simulink model "el_chem_25uA"  (R2024a)
settings: Solver=FixedStepDiscrete  StartTime=0.0  StopTime=inf  FixedStep=0.1  RelTol=1e-3
libraries: etargetslib x6, instrumentseriallib x3
settings Model: Creator=setm  LastModifiedBy=setm

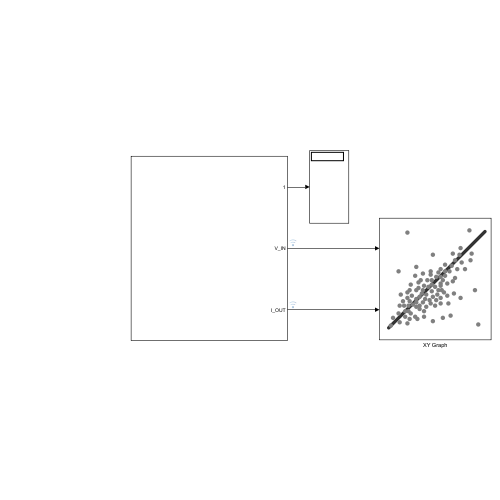
[thumbnail: Simulink's stored preview of the top-level diagram]
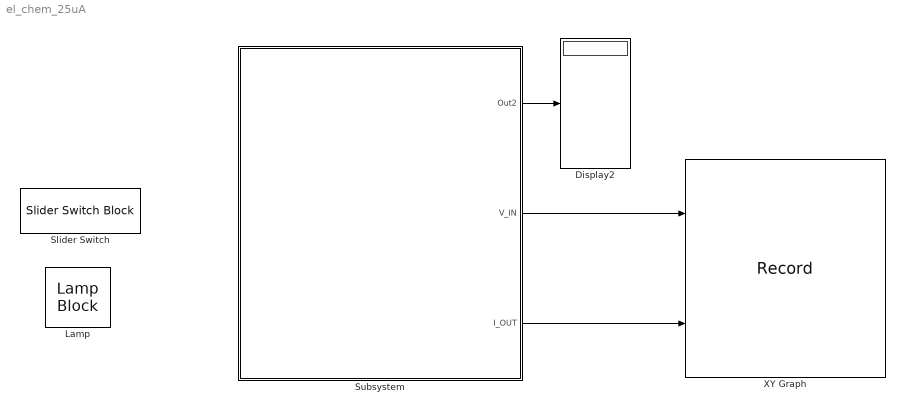
== system el_chem_25uA ==
  Display2 : Display
      settings: Decimation=5
  Lamp : LampBlock  LabelPosition=Hide
  Slider Switch : SliderSwitchBlock
      settings: Values={{'Off', 'On'}, [0 1]}
  Subsystem : Subsystem
  XY Graph : Record  FileSettingsInternal="{\"entries\":[{\"content\":{\"excelSettings\":{\"content\":{},\"type\":\"Streamout.ExcelSettings\"}},\"type\":\"Streamout.FileSettingStorage\",\"uuid\":\"\"}],\"packageUris\":[\"http:\\/\\/schema.mathworks.com\\/mf0\\/streamout_blocks\\/R2020a\"],\"version\":\"1.0\"}"  Layout=[1 1]  SignalsInternal="{\"entries\":[{\"content\":{\"signals\":[{\"content\":{\"blockPath\":[],\"dimensions\":[1],\"domain\":\"\",\"lineColor\":\"#a2142f\",\"plots\":[ 1 ],\"port\":1,\"signalID\":1,\"signalName\":\"Subsystem:2\"},\"type\":\"RecordBlkView.Signal\",\"uuid\":\"\"},{\"content\":{\"blockPath\":[],\"dimensions\":[1,1],\"domain\":\"\",\"lineColor\":\"#139fff\",\"plots\":[ 1 ],\"port\":2,\"signalID\":2,\"signalName\":\"Subsystem:3\"},\"type\":\"RecordBlkView.Signal\",\"uuid\":\"\"}]},\"type\":\"RecordBlkView.InputSignals\",\"uuid\":\"\"}],\"packageUris\":[\"http:\\/\\/schema.mathworks.com\\/mf0\\/streamout_blocks\\/R2020a\"],\"version\":\"1.0\"}"  VisualizationBindings="{\"xyplotplugin\":{\"info\":[{\"series\":[{\"bindingParametersList\":[{\"parameter\":\"X-Axis\",\"signalID\":1,\"signalName\":\"Subsystem:2\"},{\"parameter\":\"Y-Axis\",\"signalID\":2,\"signalName\":\"Subsystem:3\"}],\"seriesID\":0}],\"subplotID\":1}]}}"  CompatibilityTag=XY
  wires:
  Subsystem/1(Out2) -> Display2/1
  Subsystem/3(I_OUT) -> XY Graph/2
  Subsystem/2(V_IN) -> XY Graph/1

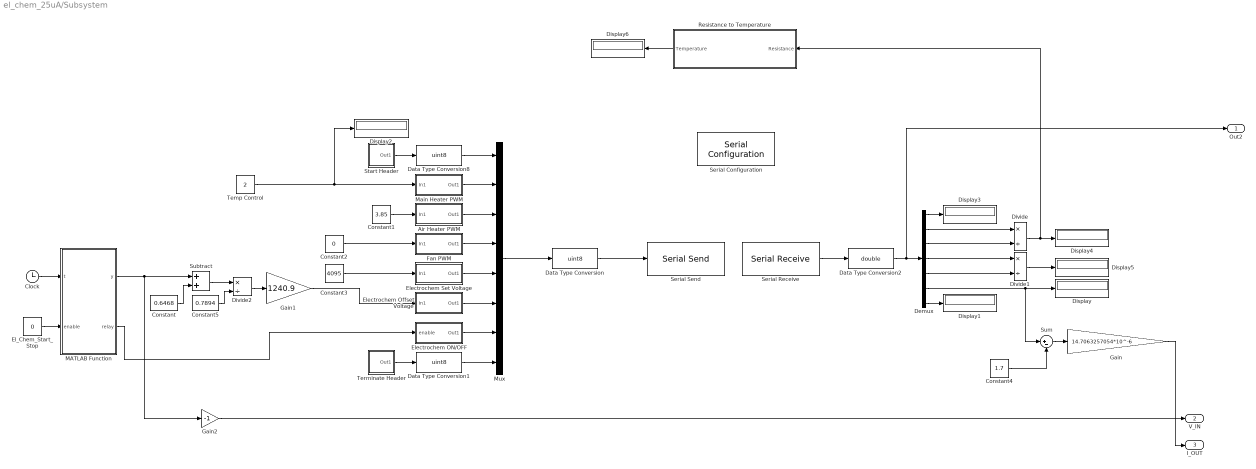
== system el_chem_25uA/Subsystem ==
  Air Heater PWM : Subsystem
  Clock : Clock
  Constant : Constant  Value=0.6468
  Constant1 : Constant  Value=3.85
  Constant2 : Constant  Value=0
  Constant3 : Constant  Value=4095
  Constant4 : Constant  Value=1.7
  Constant5 : Constant  Value=0.7894
  Data Type Conversion : DataTypeConversion  OutDataTypeStr=uint8  SaturateOnIntegerOverflow=off  RndMeth=Floor
  Data Type Conversion1 : DataTypeConversion  OutDataTypeStr=uint8  SaturateOnIntegerOverflow=off  RndMeth=Floor
  Data Type Conversion2 : DataTypeConversion  OutDataTypeStr=double  SaturateOnIntegerOverflow=off  RndMeth=Floor
  Data Type Conversion8 : DataTypeConversion  OutDataTypeStr=uint8  SaturateOnIntegerOverflow=off  RndMeth=Floor
  Demux : Demux  Outputs=7
  Display{,1..6} (7 alike) : Display
      Display1 settings: Decimation=5
      Display3 settings: Decimation=5
  Divide : Product  Inputs=*/
  Divide1 : Product  Inputs=*/
  Divide2 : Product  Inputs=*/
  El_Chem_Start_Stop : Constant  Value=0
  Electrochem ON/OFF : Subsystem
  Electrochem Offset Voltage : Subsystem
  Electrochem Set Voltage : Subsystem
  Fan PWM : Subsystem
  Gain : Gain  Gain=14.7063257054*10^-6
  Gain1 : Gain  Gain=1240.9
  Gain2 : Gain  Gain=-1
  MATLAB Function : MATLAB Function  TreatAsAtomicUnit=on
  Main Heater PWM : Subsystem
  Mux : Mux  Inputs=8
  Resistance to Temperature : Subsystem
  Serial Configuration : instrumentseriallib/Serial Configuration  Priority=-200000  PortSel=COM10  Port=COM10  ComPort=COM10  BaudRate=115200  DataBits=8  Parity=none  StopBits=1  ByteOrder=little-endian  FlowControl=none  Timeout=10  SimulateUsing=Interpreted execution  BlockInModel=on  aMode=1
  Serial Receive : instrumentseriallib/Serial Receive  Priority=1  PortSel=COM10  Port=COM10  ComPort=COM10  DataType=single  SaveDataType=uint8  ToggleHeader=off  Header=[]  ToggleDataSize=on  DataSize=[7 1]  ToggleTerminator=off  Terminator=<none>  CustomTerminator=[]  InputFormat=Column major  EnableBlockingMode=on  ActionDataUnavailable=Output last received value  ActionWhenDataUnavailable=Output last received value  CustomValue=0  SampleTime=0.1  SimulateUsing=Interpreted execution  BlockInModel=on  aMode=1
  Serial Send : instrumentseriallib/Serial Send  Priority=1  PortSel=COM10  Port=COM10  ComPort=COM10  Header=[]  Terminator=<none>  CustomTerminator=[]  EnableBlockingMode=on  SimulateUsing=Interpreted execution  BlockInModel=on  aMode=1
  Start Header : Subsystem
  Subtract : Sum
  Sum : Sum  Inputs=|+-
  Temp Control : Constant  Value=2
  Terminate Header : Subsystem
  Out2 : Outport
  V_IN : Outport  Port=2
  I_OUT : Outport  Port=3
  wires:
  Electrochem ON/OFF/1(Out1) -> Mux/7
  Constant2/1 -> Fan PWM/1(In1)
  Divide1/1 -> Display5/1
  Demux/7 -> Display1/1
  Demux/4 -> Divide1/1
  Demux/5 -> Divide1/2
  Mux/1 -> Data Type Conversion/1
  Data Type Conversion1/1 -> Mux/8
  Data Type Conversion8/1 -> Mux/1
  Data Type Conversion/1 -> Serial Send/1
  Air Heater PWM/1(Out1) -> Mux/3
  Demux/6 -> Sum/1, Display/1
  Constant1/1 -> Air Heater PWM/1(In1)
  Electrochem Offset Voltage/1(Out1) -> Mux/6
  Constant3/1 -> Electrochem Set Voltage/1(In1)
  Demux/3 -> Divide/2
  Serial Receive/1 -> Data Type Conversion2/1
  El_Chem_Start_Stop/1 -> MATLAB Function/2(enable)
  Fan PWM/1(Out1) -> Mux/4
  Divide/1 -> Resistance to Temperature/1(Resistance), Display4/1
  Electrochem Set Voltage/1(Out1) -> Mux/5
  Main Heater PWM/1(Out1) -> Mux/2
  Demux/2 -> Divide/1
  Start Header/1(Out1) -> Data Type Conversion8/1
  Resistance to Temperature/1(Temperature) -> Display6/1
  Demux/1 -> Display3/1
  Terminate Header/1(Out1) -> Data Type Conversion1/1
  Data Type Conversion2/1 -> Out2/1, Demux/1
  Temp Control/1 -> Display2/1, Main Heater PWM/1(In1)
  Clock/1 -> MATLAB Function/1(t)
  MATLAB Function/1(y) -> Subtract/1, Gain2/1
  MATLAB Function/2(relay) -> Electrochem ON/OFF/1(enable)
  Sum/1 -> Gain/1
  Constant4/1 -> Sum/2
  Gain/1 -> I_OUT/1
  Constant/1 -> Subtract/2
  Subtract/1 -> Divide2/1
  Constant5/1 -> Divide2/2
  Divide2/1 -> Gain1/1
  Gain1/1 -> Electrochem Offset Voltage/1(In1)
  Gain2/1 -> V_IN/1

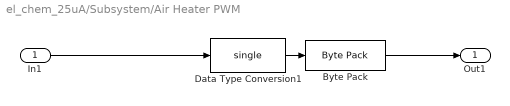
== system el_chem_25uA/Subsystem/Air Heater PWM ==
  In1 : Inport
  Byte Pack : etargetslib/Byte Pack  datatypes={'single'}  byteAlign=1
  Data Type Conversion1 : DataTypeConversion  OutDataTypeStr=single  SaturateOnIntegerOverflow=off  RndMeth=Floor
  Out1 : Outport
  wires:
  Data Type Conversion1/1 -> Byte Pack/1
  Byte Pack/1 -> Out1/1
  In1/1 -> Data Type Conversion1/1

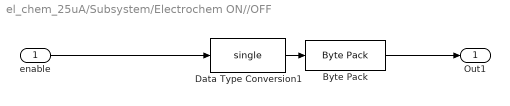
== system el_chem_25uA/Subsystem/Electrochem ON//OFF ==
  enable : Inport
  Byte Pack : etargetslib/Byte Pack  datatypes={'single'}  byteAlign=1
  Data Type Conversion1 : DataTypeConversion  OutDataTypeStr=single  SaturateOnIntegerOverflow=off  RndMeth=Floor
  Out1 : Outport
  wires:
  Data Type Conversion1/1 -> Byte Pack/1
  Byte Pack/1 -> Out1/1
  enable/1 -> Data Type Conversion1/1

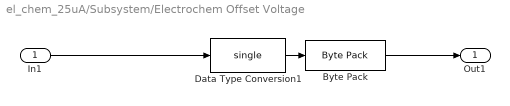
== system el_chem_25uA/Subsystem/Electrochem Offset Voltage ==
  In1 : Inport
  Byte Pack : etargetslib/Byte Pack  datatypes={'single'}  byteAlign=1
  Data Type Conversion1 : DataTypeConversion  OutDataTypeStr=single  SaturateOnIntegerOverflow=off  RndMeth=Floor
  Out1 : Outport
  wires:
  Data Type Conversion1/1 -> Byte Pack/1
  Byte Pack/1 -> Out1/1
  In1/1 -> Data Type Conversion1/1

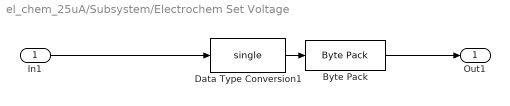
== system el_chem_25uA/Subsystem/Electrochem Set Voltage ==
  In1 : Inport
  Byte Pack : etargetslib/Byte Pack  datatypes={'single'}  byteAlign=1
  Data Type Conversion1 : DataTypeConversion  OutDataTypeStr=single  SaturateOnIntegerOverflow=off  RndMeth=Floor
  Out1 : Outport
  wires:
  Data Type Conversion1/1 -> Byte Pack/1
  Byte Pack/1 -> Out1/1
  In1/1 -> Data Type Conversion1/1

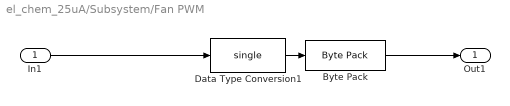
== system el_chem_25uA/Subsystem/Fan PWM ==
  In1 : Inport
  Byte Pack : etargetslib/Byte Pack  datatypes={'single'}  byteAlign=1
  Data Type Conversion1 : DataTypeConversion  OutDataTypeStr=single  SaturateOnIntegerOverflow=off  RndMeth=Floor
  Out1 : Outport
  wires:
  Data Type Conversion1/1 -> Byte Pack/1
  Byte Pack/1 -> Out1/1
  In1/1 -> Data Type Conversion1/1

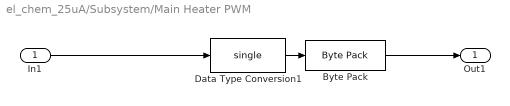
== system el_chem_25uA/Subsystem/Main Heater PWM ==
  In1 : Inport
  Byte Pack : etargetslib/Byte Pack  datatypes={'single'}  byteAlign=1
  Data Type Conversion1 : DataTypeConversion  OutDataTypeStr=single  SaturateOnIntegerOverflow=off  RndMeth=Floor
  Out1 : Outport
  wires:
  Data Type Conversion1/1 -> Byte Pack/1
  Byte Pack/1 -> Out1/1
  In1/1 -> Data Type Conversion1/1

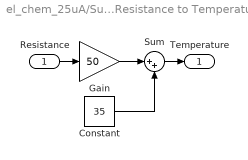
== system el_chem_25uA/Subsystem/Resistance to Temperature ==
  Resistance : Inport
  Constant : Constant  Value=35
  Gain : Gain  Gain=50
  Sum : Sum  Inputs=|++
  Temperature : Outport
  wires:
  Gain/1 -> Sum/1
  Constant/1 -> Sum/2
  Resistance/1 -> Gain/1
  Sum/1 -> Temperature/1

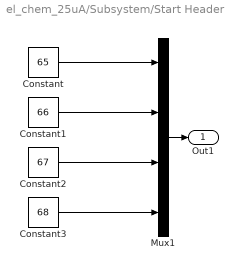
== system el_chem_25uA/Subsystem/Start Header ==
  Constant : Constant  Value=65
  Constant1 : Constant  Value=66
  Constant2 : Constant  Value=67
  Constant3 : Constant  Value=68
  Mux1 : Mux
  Out1 : Outport
  wires:
  Constant/1 -> Mux1/1
  Constant3/1 -> Mux1/4
  Constant2/1 -> Mux1/3
  Constant1/1 -> Mux1/2
  Mux1/1 -> Out1/1

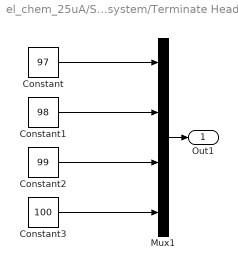
== system el_chem_25uA/Subsystem/Terminate Header ==
  Constant : Constant  Value=97
  Constant1 : Constant  Value=98
  Constant2 : Constant  Value=99
  Constant3 : Constant  Value=100
  Mux1 : Mux
  Out1 : Outport
  wires:
  Constant/1 -> Mux1/1
  Constant3/1 -> Mux1/4
  Constant2/1 -> Mux1/3
  Constant1/1 -> Mux1/2
  Mux1/1 -> Out1/1

== matlab function el_chem_25uA/Subsystem/MATLAB Function ==
  data: t input; y output; enable input; relay output
function [y, relay] = sequence_generator(t, enable)
%#codegen

% Parameters
initial_value = 0.35;
final_value = -0.15;
step_size = 0.003;
num_cycles = 6;
sample_time = 0.1;

% Calculate the number of steps
total_steps = (final_value - initial_value) / step_size;
if total_steps < 0
    total_steps = abs(total_steps);
end

% Initialize persistent variables
persistent current_value direction cycle_count step_count relay_state

if isempty(current_value)
    current_value = initial_value;
    direction = -1;  % Start by decreasing
    cycle_count = 0;
    step_count = 0;
    relay_state = 0; % Start with the relay off
end

% Output initialization
y = current_value;
relay = relay_state;

% Check if the system is enabled
if enable
    % Turn the relay on when the system starts running
    relay_state = 1;
    
    % Check if we need to update at this sample time
    if mod(t, sample_time) == 0
        % Update the value based on the direction
        if direction == -1
            current_value = current_value - step_size;
            step_count = step_count + 1;
            % Check if we have reached the final value
            if current_value <= final_value
                direction = 1; % Change direction to up
            end
        elseif direction == 1
            current_value = current_value + step_size;
            step_count = step_count + 1;
            % Check if we have reached the initial value
            if current_value >= initial_value
                direction = -1; % Change direction to down
                cycle_count = cycle_count + 1; % Complete one cycle
            end
        end
        % Reset if all cycles are complete
        if cycle_count >= num_cycles
            y = initial_value;
            relay_state = 0; % Turn off the relay when the sequence ends
            return;
        end
    end
else
    % Turn off the relay when the system is disabled
    relay_state = 0;
end

% Output the current value and relay state
y = current_value;
relay = relay_state;
end
